simulink model "demoSfun_mimo"  (R2020b)
settings: Solver=VariableStepAuto  StartTime=0.0  StopTime=10.0  RelTol=1e-3
settings Model: Creator=yinti  LastModifiedBy=yinti

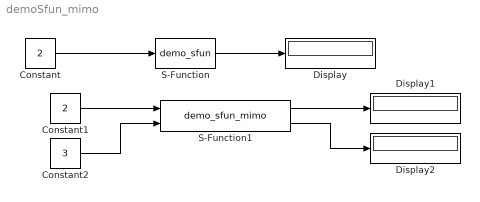
== system demoSfun_mimo ==
  Constant : Constant  Value=2
  Constant1 : Constant  Value=2
  Constant2 : Constant  Value=3
  Display : Display
  Display1 : Display
  Display2 : Display
  S-Function : S-Function  FunctionName=demo_sfun  SFunctionDeploymentMode=off  EnableBusSupport=off
  S-Function1 : S-Function  FunctionName=demo_sfun_mimo  SFunctionDeploymentMode=off  EnableBusSupport=off
  wires:
  Constant/1 -> S-Function/1
  S-Function/1 -> Display/1
  Constant1/1 -> S-Function1/1
  Constant2/1 -> S-Function1/2
  S-Function1/1 -> Display1/1
  S-Function1/2 -> Display2/1
